simulink model "problem4"  (R2020b)
settings: Solver=VariableStepAuto  StartTime=0.0  StopTime=10.0  RelTol=1e-3
settings Model: Creator=Lenovo  LastModifiedBy=Lenovo

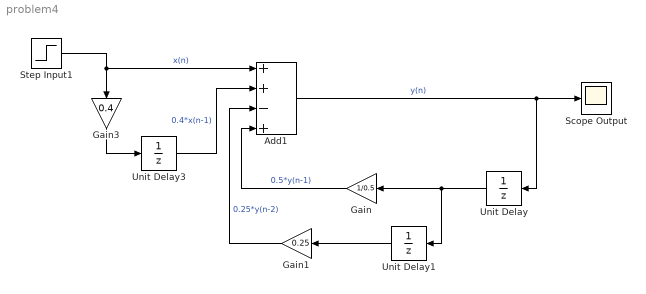
== system problem4 ==
  Add1 : Sum  Inputs=++-+
  Gain : Gain  Gain=1/0.5
  Gain1 : Gain  Gain=0.25
  Gain3 : Gain  Gain=0.4
  Scope Output : Scope
  Step Input1 : Step  SampleTime=0
  Unit Delay : UnitDelay  SampleTime=-1  HasFrameUpgradeWarning=on
  Unit Delay1 : UnitDelay  SampleTime=-1  HasFrameUpgradeWarning=on
  Unit Delay3 : UnitDelay  SampleTime=-1  HasFrameUpgradeWarning=on
  wires:
  Step Input1/1 -> Add1/1, Gain3/1  "x(n)"
  Gain3/1 -> Unit Delay3/1
  Unit Delay3/1 -> Add1/2  "0.4*x(n-1)"
  Gain/1 -> Add1/4  "0.5*y(n-1)"
  Gain1/1 -> Add1/3  "0.25*y(n-2)"
  Unit Delay/1 -> Unit Delay1/1, Gain/1
  Unit Delay1/1 -> Gain1/1
  Add1/1 -> Unit Delay/1, Scope Output/1  "y(n)"
